simulink model "problem3_simulink"  (R2017b)
settings: Solver=ode4  StartTime=0.0  StopTime=tfinal  FixedStep=h  RelTol=1e-3
libraries: cstblocks x8
settings Model: Creator=Rahul Vivek Sawant  LastModifiedBy=Rahul Vivek Sawant

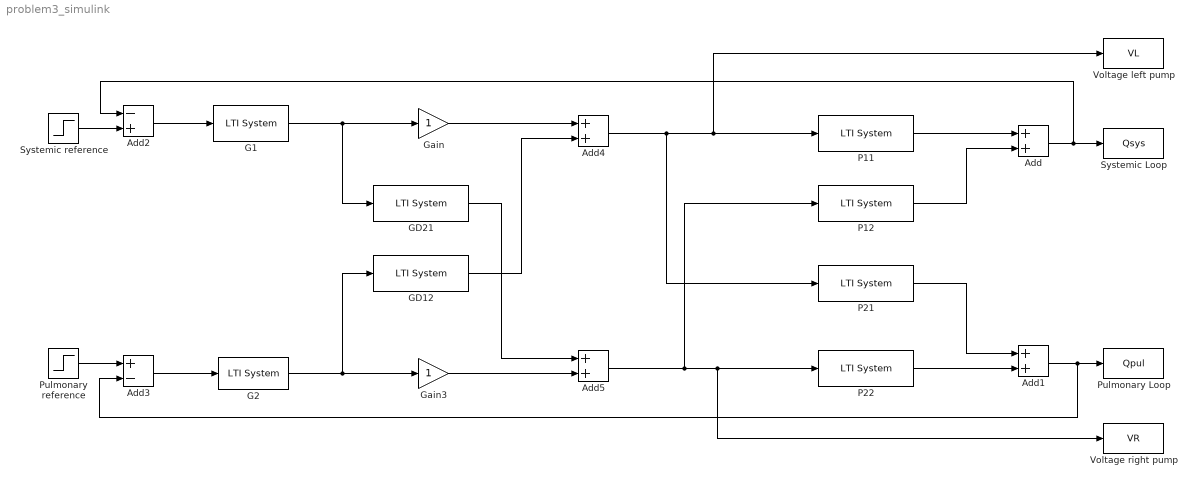
== system problem3_simulink ==
  Add{,1,4..5} (4 alike) : Sum
  Add2 : Sum  Inputs=-+
  Add3 : Sum  Inputs=+-
  G1 : cstblocks/LTI System  sys=G11  IC=[]
  G2 : cstblocks/LTI System  sys=G22  IC=[]
  GD12 : cstblocks/LTI System  sys=GD12  IC=[]
  GD21 : cstblocks/LTI System  sys=GD21  IC=[]
  Gain : Gain
  Gain3 : Gain
  P11 : cstblocks/LTI System  sys=P11  IC=[]
  P12 : cstblocks/LTI System  sys=P12  IC=[]
  P21 : cstblocks/LTI System  sys=P21  IC=[]
  P22 : cstblocks/LTI System  sys=P22  IC=[]
  Pulmonary Loop : ToWorkspace  VariableName=Qpul  SampleTime=-1
  Pulmonary reference : Step  Time=20  Before=4  After=6  SampleTime=0
  Systemic Loop : ToWorkspace  VariableName=Qsys  SampleTime=-1
  Systemic reference : Step  Time=10  Before=4  After=5  SampleTime=0
  Voltage left pump : ToWorkspace  VariableName=VL  SampleTime=-1
  Voltage right pump : ToWorkspace  VariableName=VR  SampleTime=-1
  wires:
  Systemic reference/1 -> Add2/2
  Pulmonary reference/1 -> Add3/1
  P21/1 -> Add1/1
  Add3/1 -> G2/1
  P22/1 -> Add1/2
  Add1/1 -> Add3/2, Pulmonary Loop/1
  GD21/1 -> Add5/1
  Add4/1 -> P21/1, Voltage left pump/1, P11/1
  Add/1 -> Add2/1, Systemic Loop/1
  G1/1 -> Gain/1, GD21/1
  P11/1 -> Add/1
  Gain3/1 -> Add5/2
  Gain/1 -> Add4/1
  P12/1 -> Add/2
  G2/1 -> Gain3/1, GD12/1
  GD12/1 -> Add4/2
  Add5/1 -> P12/1, Voltage right pump/1, P22/1
  Add2/1 -> G1/1
